simulink model "BLCTRL"  (R2020b)
settings: Solver=FixedStepAuto  StartTime=0.0  StopTime=TMax  FixedStep=DT  RelTol=1e-3  EnableMultiTasking=on
undefined symbols (not defined in the file or in its folder): BLCTRL_K_I, BLCTRL_K_P, BLCTRL_K_T, BLCTRL_KK, BLCTRL_M_1, BLCTRL_M_2, BLCTRL_Omega_1, BLCTRL_Omega_2, BLCTRL_Omega_rated, BLCTRL_P_rated, BLCTRL_T, BLCTRL_theta_max, BLCTRL_theta_rate, BLCTRL_theta_star, BLCTRL_theta_sw, BLCTRL_torque_rate, DiscIntNeverNeededParam
settings Model: Creator=lpwoolcock  LastModifiedBy=lukew

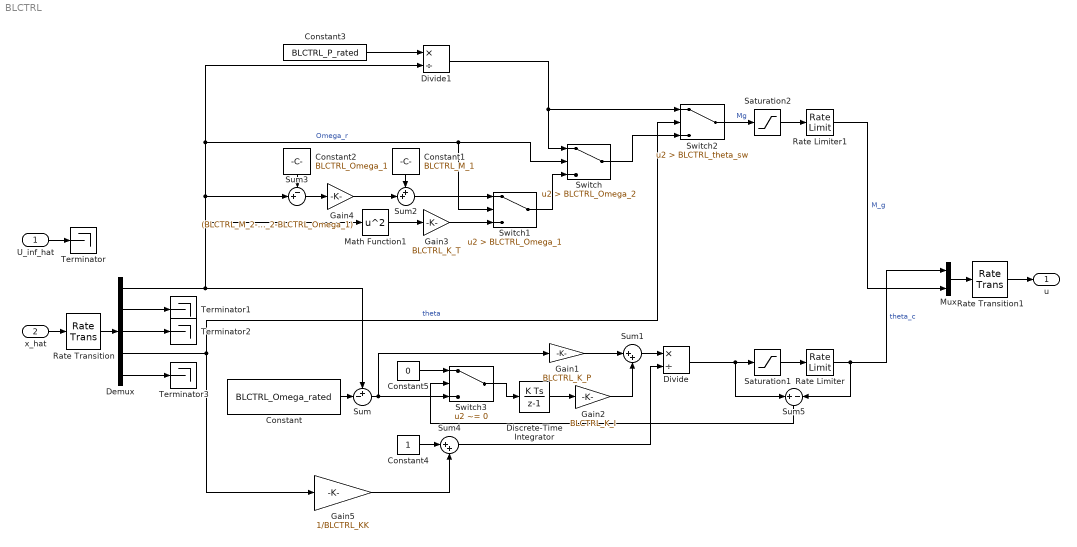
== system BLCTRL ==
  U_inf_hat : Inport  PortDimensions=1
  x_hat : Inport  Port=2  PortDimensions=[5 1]
  Constant : Constant  Value=BLCTRL_Omega_rated  SampleTime=BLCTRL_T
  Constant1 : Constant  Value=BLCTRL_M_1  SampleTime=BLCTRL_T
  Constant2 : Constant  Value=BLCTRL_Omega_1  SampleTime=BLCTRL_T
  Constant3 : Constant  Value=BLCTRL_P_rated  SampleTime=BLCTRL_T
  Constant4 : Constant  SampleTime=BLCTRL_T
  Constant5 : Constant  Value=0  SampleTime=BLCTRL_T
  Demux : Demux  Outputs=5
  Discrete-Time Integrator : DiscreteIntegrator  SampleTime=BLCTRL_T  ICPrevOutput=DiscIntNeverNeededParam  ICPrevScaledInput=DiscIntNeverNeededParam
  Divide : Product  Inputs=*/
  Divide1 : Product  Inputs=*/
  Gain1 : Gain  Gain=BLCTRL_K_P
  Gain2 : Gain  Gain=BLCTRL_K_I
  Gain3 : Gain  Gain=BLCTRL_K_T
  Gain4 : Gain  Gain=(BLCTRL_M_2-BLCTRL_M_1)/(BLCTRL_Omega_2-BLCTRL_Omega_1)
  Gain5 : Gain  Gain=1/BLCTRL_KK
  Math Function1 : Math  Operator=square  SaturateOnIntegerOverflow=on
  Mux : Mux  Inputs=2
  Rate Limiter : RateLimiter  RisingSlewLimit=BLCTRL_theta_rate  FallingSlewLimit=-BLCTRL_theta_rate  SampleTimeMode=inherited
  Rate Limiter1 : RateLimiter  RisingSlewLimit=BLCTRL_torque_rate  FallingSlewLimit=-BLCTRL_torque_rate  SampleTimeMode=inherited
  Rate Transition : RateTransition  InitialCondition=zeros(5,1)  OutPortSampleTime=BLCTRL_T
  Rate Transition1 : RateTransition  InitialCondition=zeros(2,1)
  Saturation1 : Saturate  UpperLimit=BLCTRL_theta_max  LowerLimit=BLCTRL_theta_star
  Saturation2 : Saturate  UpperLimit=1.1*BLCTRL_M_2  LowerLimit=-1.1*BLCTRL_M_2
  Sum : Sum  Inputs=+-|
  Sum1 : Sum  Inputs=|++
  Sum2 : Sum  Inputs=++|
  Sum3 : Sum  Inputs=-+|
  Sum4 : Sum  Inputs=|++
  Sum5 : Sum  Inputs=+|-
  Switch : Switch  Criteria=u2 > Threshold  Threshold=BLCTRL_Omega_2
  Switch1 : Switch  Criteria=u2 > Threshold  Threshold=BLCTRL_Omega_1
  Switch2 : Switch  Criteria=u2 > Threshold  Threshold=BLCTRL_theta_sw
  Switch3 : Switch  Criteria=u2 ~= 0  Threshold=BLCTRL_Omega_1
  Terminator{,1..3} (4 alike) : Terminator
  u : Outport  PortDimensions=[2 1]
  wires:
  Constant/1 -> Sum/2
  Gain1/1 -> Sum1/1
  Discrete-Time Integrator/1 -> Gain2/1
  Switch1/1 -> Switch/3
  Gain3/1 -> Switch1/3
  Math Function1/1 -> Gain3/1
  Sum2/1 -> Switch1/1
  Constant1/1 -> Sum2/1
  Gain4/1 -> Sum2/2
  Sum3/1 -> Gain4/1
  Constant2/1 -> Sum3/1
  Mux/1 -> Rate Transition1/1
  x_hat/1 -> Rate Transition/1
  Demux/4 -> Switch2/2, Gain5/1  "theta"
  Demux/1 -> Math Function1/1, Sum3/2, Switch1/2, Switch/2, Divide1/2, Sum/1  "Omega_r"
  Demux/5 -> Terminator3/1
  Demux/3 -> Terminator2/1
  Demux/2 -> Terminator1/1
  U_inf_hat/1 -> Terminator/1
  Gain5/1 -> Sum4/2
  Constant4/1 -> Sum4/1
  Gain2/1 -> Sum1/2
  Sum1/1 -> Divide/1
  Divide/1 -> Sum5/1, Saturation1/1
  Sum4/1 -> Divide/2
  Saturation1/1 -> Rate Limiter/1
  Rate Limiter/1 -> Sum5/2, Mux/1  "theta_c"
  Constant3/1 -> Divide1/1
  Divide1/1 -> Switch2/1, Switch/1
  Switch/1 -> Switch2/3
  Switch2/1 -> Saturation2/1  "Mg"
  Saturation2/1 -> Rate Limiter1/1
  Rate Limiter1/1 -> Mux/2  "M_g"
  Sum/1 -> Switch3/3, Gain1/1
  Switch3/1 -> Discrete-Time Integrator/1
  Constant5/1 -> Switch3/1
  Sum5/1 -> Switch3/2
  Rate Transition/1 -> Demux/1
  Rate Transition1/1 -> u/1
